simulink model "Punto4"  (R2022a)
settings: Solver=VariableStepAuto  StartTime=0.0  StopTime=700  RelTol=1e-3
undefined symbols (not defined in the file or in its folder): B1, beta, k, m1, r1, r2, t1, t2
settings Model: Creator=juand  LastModifiedBy=juand

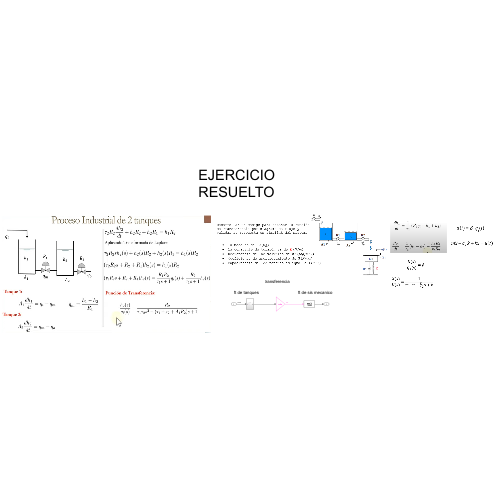
[thumbnail: Simulink's stored preview of the top-level diagram]
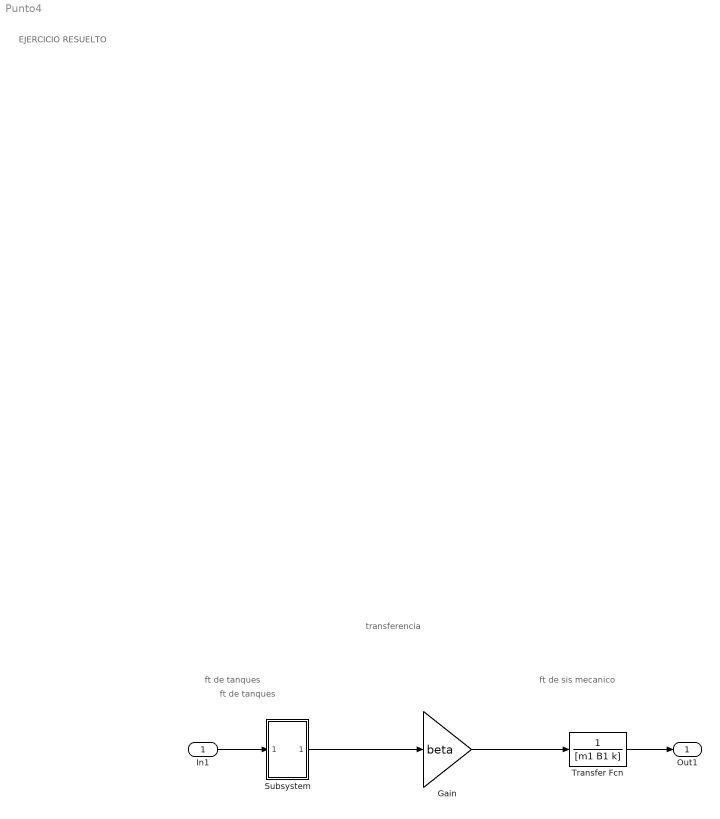
== system Punto4 ==
  note: EJERCICIO RESUELTO
  note: ft de tanques
  note: ft de tanques
  note: transferencia
  note: ft de sis mecanico
  In1 : Inport
  Gain : Gain  Gain=beta
  Subsystem : Subsystem
  Transfer Fcn : TransferFcn  Denominator=[m1 B1 k]
  Out1 : Outport
  wires:
  Gain/1 -> Transfer Fcn/1
  In1/1 -> Subsystem/1(In1)
  Subsystem/1(Out1) -> Gain/1
  Transfer Fcn/1 -> Out1/1

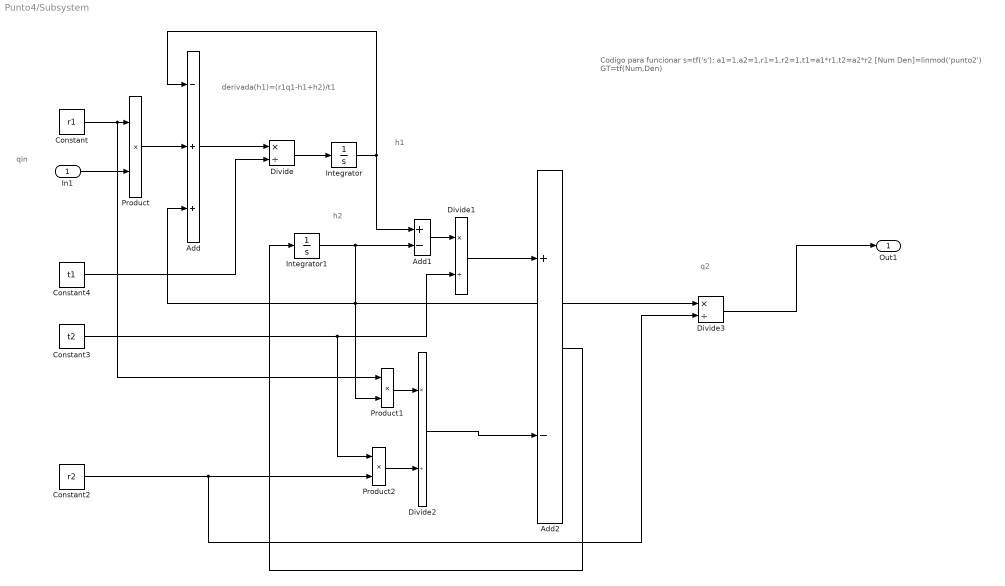
== system Punto4/Subsystem ==
  note: Codigo para funcionar
      | s=tf('s');
      | a1=1,a2=1,r1=1,r2=1,t1=a1*r1,t2=a2*r2
      | [Num Den]=linmod('punto2')
      | GT=tf(Num,Den)
  note: h1
  note: derivada(h1)=(r1q1-h1+h2)/t1
  note: h2
  note: q2
  note: qin
  In1 : Inport
  Add : Sum  Inputs=-++
  Add1 : Sum  Inputs=+-
  Add2 : Sum  Inputs=+-
  Constant : Constant  Value=r1
  Constant2 : Constant  Value=r2
  Constant3 : Constant  Value=t2
  Constant4 : Constant  Value=t1
  Divide{,1..3} (4 alike) : Product  Inputs=*/
  Integrator : Integrator
  Integrator1 : Integrator
  Product : Product
  Product1 : Product
  Product2 : Product
  Out1 : Outport
  wires:
  Product2/1 -> Divide2/2
  In1/1 -> Product/2
  Integrator/1 -> Add/1, Add1/1
  Constant/1 -> Product1/1, Product/1
  Product/1 -> Add/2
  Constant2/1 -> Divide3/2, Product2/2
  Constant3/1 -> Product2/1, Divide1/2
  Constant4/1 -> Divide/2
  Divide/1 -> Integrator/1
  Add/1 -> Divide/1
  Add2/1 -> Integrator1/1
  Add1/1 -> Divide1/1
  Product1/1 -> Divide2/1
  Divide2/1 -> Add2/2
  Divide1/1 -> Add2/1
  Divide3/1 -> Out1/1
  Integrator1/1 -> Add1/2, Add/3, Product1/2, Divide3/1
